simulink model "simulacion"  (R2021a)
settings: Solver=VariableStepAuto  StartTime=0.0  StopTime=10.0  RelTol=1e-3
values from neighbouring files (symbols this model uses):
  Gm1 = tf(tf1.numerator/tf1.denominator(end),tf1.denominator/tf1.denominator(end))    [desarrollo.m]
  Gm2 = tf(tf2.numerator/tf2.denominator(end),tf2.denominator/tf2.denominator(end))    [desarrollo.m]
  Gm3 = tf(tf3.numerator/tf3.denominator(end),tf3.denominator/tf3.denominator(end))    [desarrollo.m]
  Kp1 = -polyval(Gm1.den{1},polo_des)/polyval(Gm1.num{1},polo_des)    [desarrollo.m]
  Kp2 = -polyval(Gm2.den{1},polo_des)/polyval(Gm2.num{1},polo_des)    [desarrollo.m]
  Kp3 = -polyval(Gm3.den{1},polo_des)/polyval(Gm3.num{1},polo_des)    [desarrollo.m]
settings Model: Creator=pierr  LastModifiedBy=pierr

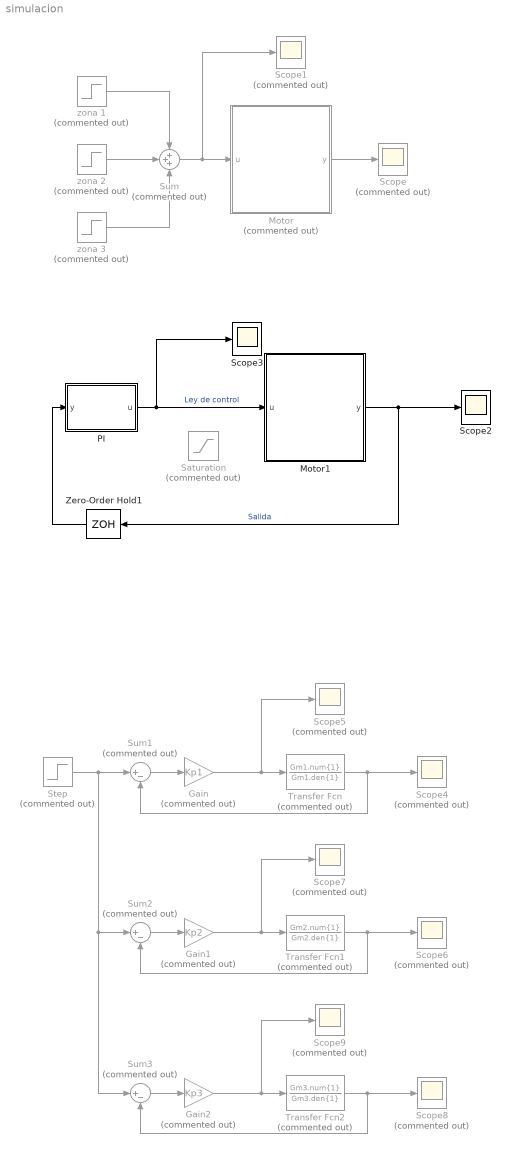
== system simulacion ==
  Gain : Gain  Commented=on  Gain=Kp1
  Gain1 : Gain  Commented=on  Gain=Kp2
  Gain2 : Gain  Commented=on  Gain=Kp3
  Motor : Subsystem  Commented=on
  Motor1 : Subsystem
  PI : MATLAB Function  TreatAsAtomicUnit=on
  Saturation : Saturate  Commented=on  UpperLimit=4  LowerLimit=-4
  Scope{,1,4..9} (8 alike) : Scope  Commented=on
  Scope2 : Scope
  Scope3 : Scope
  Step : Step  Commented=on  Time=0  After=180  SampleTime=0
  Sum : Sum  Commented=on  Inputs=+++
  Sum1 : Sum  Commented=on  Inputs=|+-
  Sum2 : Sum  Commented=on  Inputs=|+-
  Sum3 : Sum  Commented=on  Inputs=|+-
  Transfer Fcn : TransferFcn  Commented=on  Numerator=Gm1.num{1}  Denominator=Gm1.den{1}
  Transfer Fcn1 : TransferFcn  Commented=on  Numerator=Gm2.num{1}  Denominator=Gm2.den{1}
  Transfer Fcn2 : TransferFcn  Commented=on  Numerator=Gm3.num{1}  Denominator=Gm3.den{1}
  Zero-Order Hold1 : ZeroOrderHold  SampleTime=0.006
  zona 1 : Step  Commented=on  Time=0  After=-3.5  SampleTime=0
  zona 2 : Step  Commented=on  Time=2  After=2  SampleTime=0
  zona 3 : Step  Commented=on  Time=4  After=3.5  SampleTime=0
  wires:
  Motor/1(y) -> Scope/1
  zona 1/1 -> Sum/1
  zona 2/1 -> Sum/2
  zona 3/1 -> Sum/3
  Sum/1 -> Scope1/1, Motor/1(u)
  Motor1/1(y) -> Zero-Order Hold1/1, Scope2/1  "Salida"
  Zero-Order Hold1/1 -> PI/1(y)
  PI/1(u) -> Scope3/1, Motor1/1(u)  "Ley de control"
  Step/1 -> Sum3/1, Sum2/1, Sum1/1
  Sum1/1 -> Gain/1
  Gain/1 -> Scope5/1, Transfer Fcn/1
  Transfer Fcn/1 -> Scope4/1, Sum1/2
  Transfer Fcn1/1 -> Scope6/1, Sum2/2
  Sum2/1 -> Gain1/1
  Gain1/1 -> Scope7/1, Transfer Fcn1/1
  Transfer Fcn2/1 -> Scope8/1, Sum3/2
  Sum3/1 -> Gain2/1
  Gain2/1 -> Scope9/1, Transfer Fcn2/1

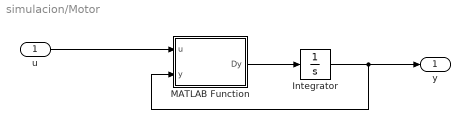
== system simulacion/Motor ==
  u : Inport
  Integrator : Integrator
  MATLAB Function : MATLAB Function  TreatAsAtomicUnit=on
  y : Outport
  wires:
  u/1 -> MATLAB Function/1(u)
  MATLAB Function/1(Dy) -> Integrator/1
  Integrator/1 -> MATLAB Function/2(y), y/1

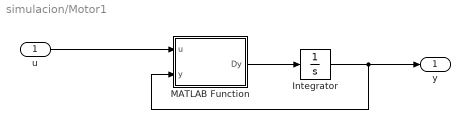
== system simulacion/Motor1 ==
  u : Inport
  Integrator : Integrator
  MATLAB Function : MATLAB Function  TreatAsAtomicUnit=on
  y : Outport
  wires:
  u/1 -> MATLAB Function/1(u)
  MATLAB Function/1(Dy) -> Integrator/1
  Integrator/1 -> MATLAB Function/2(y), y/1

== matlab function simulacion/Motor/MATLAB Function ==
  data: u input; Dy output; y input
function Dy = fcn(u,y)
%#codegen
if u>=-4 &&u<=-3
    K=110.6;
    tau=0.02982;
elseif u>-3 && u<=-0
    K=109.8;
    tau=0.02589;
elseif u>0 &&u<=4
    K=113.6;
    tau=0.02975;
else
    Dy=0;
    return
end
Dy = (K*u-y)/tau;

== matlab function simulacion/PI ==
  data: y input; u output
function u = fcn(y)

r=-180;%establecer referencia

persistent u_1
persistent e_1
if isempty(u_1)
    u_1=0;
    e_1=0;
end
e=r-y;
Ts=0.006;
if u_1>=-4 && u_1<=-3
    Kp=0.006960088061646;
    Ki=0.055680704493166;
elseif u_1>-3 && u_1<=-0
    Kp=0.007628282118139;
    Ki=0.061026256945111;
elseif u_1>0 &&u_1<=4
    Kp=0.007214135537514;
    Ki=0.057713084300112;
else
    Kp=0;
    Ki=0;
end
u=u_1+(2*Kp+Ki*Ts)/2*e+(Ki*Ts-2*Kp)/2*e_1;
if u<-4
    u=-4;
elseif u>4
    u=4;
end
e_1=e;
u_1=u;

== matlab function simulacion/Motor1/MATLAB Function ==
  data: u input; Dy output; y input
function Dy = fcn(u,y)
%#codegen
if u<=-3
    K=110.6;
    tau=0.02982;
elseif u>-3 && u<=-0
    K=109.8;
    tau=0.02589;
else
    K=113.6;
    tau=0.02975;
end
Dy = (K*u-y)/tau;
